simulink model "ball_beam_model_complete"  (R2014a)
settings: Solver=ode45  StartTime=0.0  StopTime=10.0  RelTol=1e-3
settings Model: Creator=Wolfgang  LastModifiedBy=Wolfgang

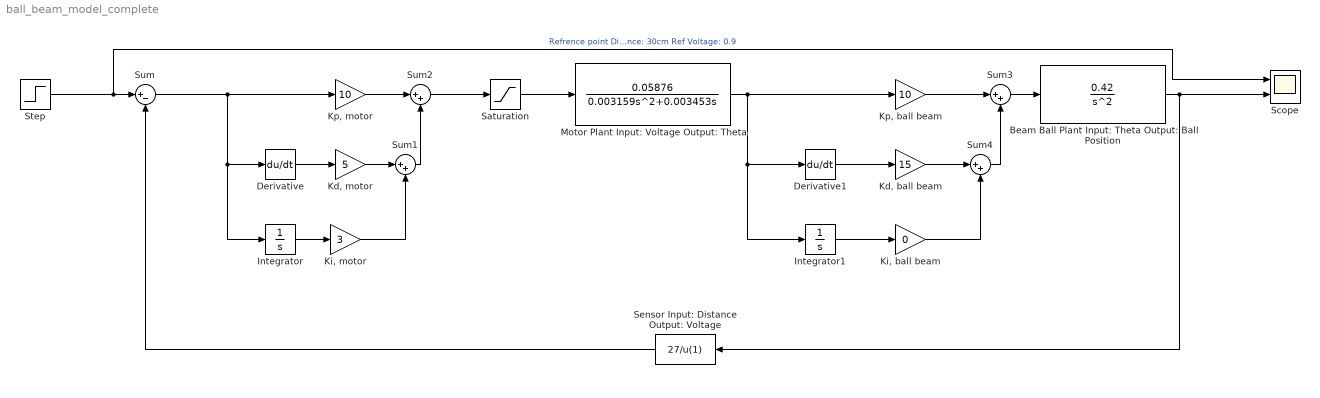
== system ball_beam_model_complete ==
  Beam Ball Plant Input: Theta Output: Ball Position : TransferFcn  Numerator=[0.42]  Denominator=[1 0 0]
  Derivative : Derivative
  Derivative1 : Derivative
  Integrator : Integrator
  Integrator1 : Integrator
  "Kd, ball beam" : Gain  Gain=15
  "Kd, motor" : Gain  Gain=5
  "Ki, ball beam" : Gain  Gain=0
  "Ki, motor" : Gain  Gain=3
  "Kp, ball beam" : Gain  Gain=10
  "Kp, motor" : Gain  Gain=10
  Motor Plant Input: Voltage Output: Theta : TransferFcn  Numerator=[0.05876]  Denominator=[0.003159 0.003453 0]
  Saturation : Saturate  UpperLimit=24  LowerLimit=-24
  Scope : Scope  NumInputPorts=2
      settings: YMin=-5~-5  YMax=5~5
  Sensor Input: Distance Output: Voltage : Fcn  Expr=27/u(1)
  Step : Step  After=0.9  SampleTime=0
  Sum : Sum  Inputs=|+-
  Sum{1..4} (4 alike) : Sum  Inputs=|++
  wires:
  Step/1 -> Scope/1, Sum/1  "Refrence point Distance: 30cm Ref Voltage: 0.9"
  "Kd, motor"/1 -> Sum1/1
  "Ki, motor"/1 -> Sum1/2
  Integrator/1 -> "Ki, motor"/1
  Derivative/1 -> "Kd, motor"/1
  Sum1/1 -> Sum2/2
  "Kp, motor"/1 -> Sum2/1
  Sum/1 -> Integrator/1, Derivative/1, "Kp, motor"/1
  Integrator1/1 -> "Ki, ball beam"/1
  Derivative1/1 -> "Kd, ball beam"/1
  "Ki, ball beam"/1 -> Sum4/2
  "Kd, ball beam"/1 -> Sum4/1
  Sum4/1 -> Sum3/2
  Sum3/1 -> Beam Ball Plant Input: Theta Output: Ball Position/1
  "Kp, ball beam"/1 -> Sum3/1
  Motor Plant Input: Voltage Output: Theta/1 -> Derivative1/1, Integrator1/1, "Kp, ball beam"/1
  Saturation/1 -> Motor Plant Input: Voltage Output: Theta/1
  Sum2/1 -> Saturation/1
  Beam Ball Plant Input: Theta Output: Ball Position/1 -> Scope/2, Sensor Input: Distance Output: Voltage/1
  Sensor Input: Distance Output: Voltage/1 -> Sum/2
